simulink model "Pendulum_VariantNew_Val"  (R2025b)
settings: Solver=VariableStepAuto  StartTime=0.0  StopTime=30  RelTol=1e-3
settings Model: Creator=djangovanderplas  LastModifiedBy=djangovanderplas

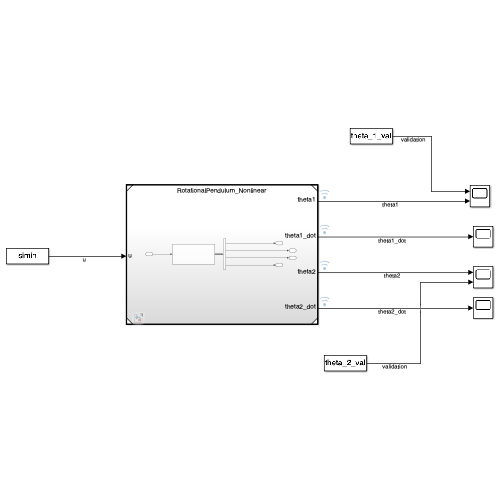
[thumbnail: Simulink's stored preview of the top-level diagram]
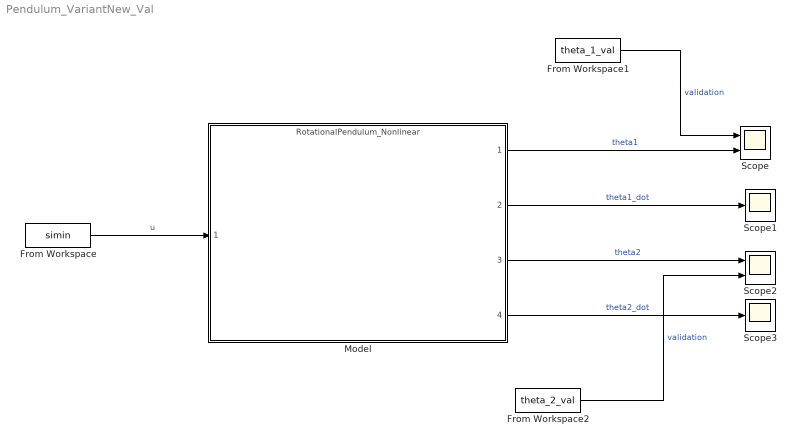
== system Pendulum_VariantNew_Val ==
  From Workspace : FromWorkspace  VariableName=simin
  From Workspace1 : FromWorkspace  VariableName=theta_1_val
  From Workspace2 : FromWorkspace  VariableName=theta_2_val
  Model : ModelReference  ModelNameDialog=RotationalPendulum_Nonlinear.slx  SimulationMode=Normal  ModelReferenceVersion=1.11
  Scope : Scope  NumInputPorts=2
      settings: ActiveDisplayYMinimum=2.2876166993214198  ActiveDisplayYMaximum=3.7574150588595887
  Scope1 : Scope
      settings: ActiveDisplayYMinimum=-1  ActiveDisplayYMaximum=1
  Scope2 : Scope  NumInputPorts=2
      settings: ActiveDisplayYMinimum=-1.3106669758287322  ActiveDisplayYMaximum=1.5804728711958125  DataLoggingVariableName=ScopeData2
  Scope3 : Scope
      settings: ActiveDisplayYMinimum=-1  ActiveDisplayYMaximum=1  DataLoggingVariableName=ScopeData3
  wires:
  Model/1 -> Scope/2  "theta1"
  Model/2 -> Scope1/1  "theta1_dot"
  Model/3 -> Scope2/1  "theta2"
  Model/4 -> Scope3/1  "theta2_dot"
  From Workspace/1 -> Model/1  "u"
  From Workspace1/1 -> Scope/1  "validation"
  From Workspace2/1 -> Scope2/2  "validation"
